simulink model "arq1"  (R2013a)
settings: Solver=ode45  StartTime=0.0  StopTime=Tsim  RelTol=1e-3
values from neighbouring files (symbols this model uses):
  D = 4.1019    [load_variables.m]    (also in matlab.mat; matlab2.mat; matlab_workspace.mat)
  dist = 5    [load_variables.m]    (also in matlab.mat; matlab2.mat; matlab_workspace.mat)
  I = 0.0044    [load_variables.m]    (also in matlab.mat; matlab2.mat; matlab_workspace.mat)
  P = 0.3105    [load_variables.m]    (also in matlab.mat; matlab2.mat; matlab_workspace.mat)
  ref = 10    [load_variables.m]    (also in matlab.mat; matlab2.mat; matlab_workspace.mat)
  Tdist = Tstep    [RenameVar.m]    (also in matlab.mat = 1200; matlab2.mat = 1200; matlab_workspace.mat = 1400)
  Tdistdown = Tstepdown    [RenameVar.m]    (also in matlab.mat = 1800; matlab2.mat = 1800; matlab_workspace.mat = 1800)
  Tref = 800    [load_variables.m]    (also in matlab.mat = 600; matlab2.mat = 600; matlab_workspace.mat = 700)
  Trefdown = Tref+Tstepdown    (= 2420)    [load_variables.m]    (also in matlab.mat = 2400; matlab2.mat = 2400; matlab_workspace.mat = 2500)
  Ts = 5    [load_variables.m]    (also in matlab.mat; matlab2.mat; matlab_workspace.mat)
  Tsim = Tref+Trefdown    (= 3220)    [load_variables.m]    (also in matlab.mat = 800; matlab2.mat = 800; matlab_workspace.mat = 3200)
libraries: opclib x3, simulink x2, commchan3 x1, cstblocks x1
settings Model: Creator=didaticontrol  LastModifiedBy=didaticontrol

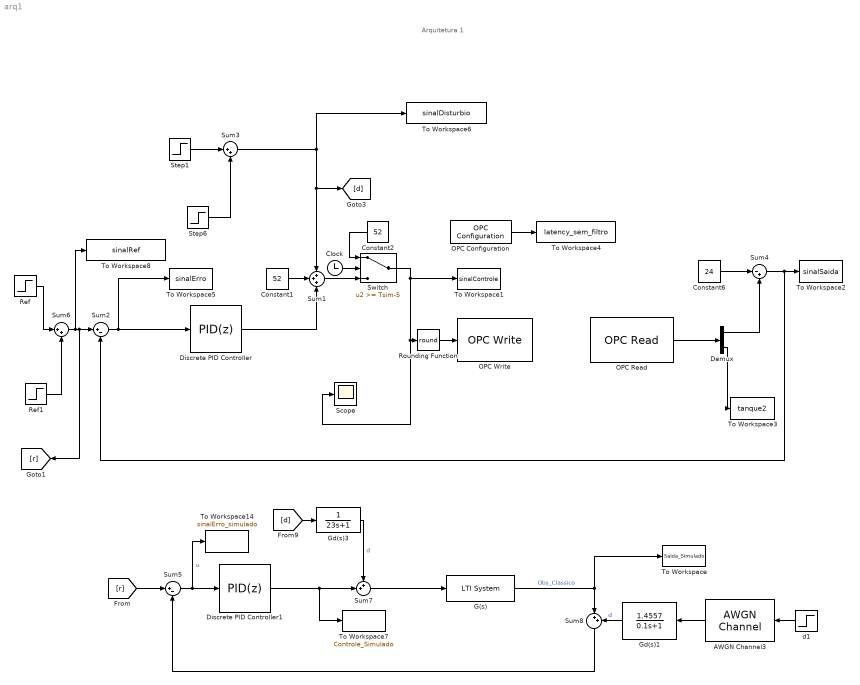
== system arq1 ==
  note: Arquitetura 1
  AWGN Channel3 : commchan3/AWGN Channel  InputProcessing=Columns as channels (frame based)  seed=67  noiseMode=Variance from mask  EbNodB=10  EsNodB=10  SNRdB=10  bitsPerSym=1  Ps=1  Tsym=1  variance=var_ruido
  Clock : Clock
  Constant1 : Constant  Value=52
  Constant2 : Constant  Value=52
  Constant6 : Constant  Value=24
  Demux : Demux  Outputs=2
  Discrete PID Controller : simulink/Continuous/PID Controller  Controller=PID  TimeDomain=Discrete-time  SampleTime=Ts  IntegratorMethod=Forward Euler  FilterMethod=Forward Euler  Form=Parallel  P=P  I=I  D=D  N=0  InitialConditionSource=internal  InitialConditionForIntegrator=0  InitialConditionForFilter=0  ExternalReset=none  LimitOutput=off  UpperSaturationLimit=inf  LowerSaturationLimit=-inf  LinearizeAsGain=off  AntiWindupMode=none  Kb=1  TrackingMode=off  Kt=1  PParamMin=[]  PParamMax=[]  IParamMin=[]  IParamMax=[]  DParamMin=[]  DParamMax=[]  NParamMin=[]  NParamMax=[]  KbParamMin=[]  KbParamMax=[]  KtParamMin=[]  KtParamMax=[]  POutMin=[]  POutMax=[]  IOutMin=[]  IOutMax=[]  DOutMin=[]  DOutMax=[]  NOutMin=[]  NOutMax=[]  KbOutMin=[]  KbOutMax=[]  KtOutMin=[]  KtOutMax=[]  IntegratorOutMin=[]  IntegratorOutMax=[]  FilterOutMin=[]  FilterOutMax=[]  SumOutMin=[]  SumOutMax=[]  SumI1OutMin=[]  SumI1OutMax=[]  SumI2OutMin=[]  SumI2OutMax=[]  SumI3OutMin=[]  SumI3OutMax=[]  SumDOutMin=[]  SumDOutMax=[]  SaturationOutMin=[]  SaturationOutMax=[]  IntegratorContinuousStateAttributes=''  IntegratorStateMustResolveToSignalObject=off  IntegratorRTWStateStorageClass=Auto  FilterContinuousStateAttributes=''  FilterStateMustResolveToSignalObject=off  FilterRTWStateStorageClass=Auto
  Discrete PID Controller1 : simulink/Continuous/PID Controller  Controller=PID  TimeDomain=Discrete-time  SampleTime=Ts  IntegratorMethod=Forward Euler  FilterMethod=Forward Euler  Form=Parallel  P=P  I=I  D=D  N=0  InitialConditionSource=internal  InitialConditionForIntegrator=0  InitialConditionForFilter=0  ExternalReset=none  LimitOutput=off  UpperSaturationLimit=inf  LowerSaturationLimit=-inf  LinearizeAsGain=off  AntiWindupMode=none  Kb=1  TrackingMode=off  Kt=1  PParamMin=[]  PParamMax=[]  IParamMin=[]  IParamMax=[]  DParamMin=[]  DParamMax=[]  NParamMin=[]  NParamMax=[]  KbParamMin=[]  KbParamMax=[]  KtParamMin=[]  KtParamMax=[]  POutMin=[]  POutMax=[]  IOutMin=[]  IOutMax=[]  DOutMin=[]  DOutMax=[]  NOutMin=[]  NOutMax=[]  KbOutMin=[]  KbOutMax=[]  KtOutMin=[]  KtOutMax=[]  IntegratorOutMin=[]  IntegratorOutMax=[]  FilterOutMin=[]  FilterOutMax=[]  SumOutMin=[]  SumOutMax=[]  SumI1OutMin=[]  SumI1OutMax=[]  SumI2OutMin=[]  SumI2OutMax=[]  SumI3OutMin=[]  SumI3OutMax=[]  SumDOutMin=[]  SumDOutMax=[]  SaturationOutMin=[]  SaturationOutMax=[]  IntegratorContinuousStateAttributes=''  IntegratorStateMustResolveToSignalObject=off  IntegratorRTWStateStorageClass=Auto  FilterContinuousStateAttributes=''  FilterStateMustResolveToSignalObject=off  FilterRTWStateStorageClass=Auto
  G(s) : cstblocks/LTI System  sys=Gs  IC=[]
  Gd(s)1 : TransferFcn  Numerator=1.4557  Denominator=[0.1 1]
  Gd(s)3 : TransferFcn  Numerator=1  Denominator=[23 1]
  OPC Configuration : opclib/OPC Configuration  opcServers=143.106.123.105/BR.OPC.Server_AR/10  errMissingItems=Error  errReadWrite=Warn  errShutdown=Error  errRTViolation=Warn  rtEnable=on  speedup=1  showLatency=on  beingUsed=on
  OPC Read : opclib/OPC Read  serverHost=143.106.123.105  serverID=BR.OPC.Server_AR  itemIDs=PTQ4_corrigido, PTQ2_corrigido  readMode=Synchronous (cache)  dataType=double  updateRate=5  showQual=off  showTS=off  tsMode=Seconds since start
  OPC Write : opclib/OPC Write  serverHost=143.106.123.105  serverID=BR.OPC.Server_AR  itemIDs=Bomba2  writeMode=Synchronous  updateRate=-1
  Ref : Step  Time=Tref  After=ref  SampleTime=0
  Ref1 : Step  Time=Trefdown  After=-ref  SampleTime=0
  Rounding Function : Rounding  Operator=round
  Scope : Scope
      settings: YMin=59.0892  YMax=59.0892
  Step1 : Step  Time=Tdist  After=dist  SampleTime=0
  Step6 : Step  Time=Tdistdown  After=-dist  SampleTime=0
  Sum1 : Sum  Inputs=+++
  Sum2 : Sum  Inputs=|+-
  Sum3 : Sum  Inputs=|++
  Sum4 : Sum  Inputs=|-+
  Sum5 : Sum  Inputs=|+-
  Sum6 : Sum  Inputs=|++
  Sum7 : Sum  Inputs=++|
  Sum8 : Sum  Inputs=|++
  Switch : Switch  Threshold=Tsim-5
  To Workspace : ToWorkspace  VariableName=Saida_Simulado  SampleTime=-1  SaveFormat=Timeseries
  To Workspace1 : ToWorkspace  VariableName=sinalControle  SampleTime=Ts  SaveFormat=Timeseries
  To Workspace14 : ToWorkspace  VariableName=sinalErro_simulado  SampleTime=Ts  SaveFormat=Timeseries
  To Workspace2 : ToWorkspace  VariableName=sinalSaida  SampleTime=Ts  SaveFormat=Timeseries
  To Workspace3 : ToWorkspace  VariableName=tanque2  SampleTime=Ts  SaveFormat=Timeseries
  To Workspace4 : ToWorkspace  VariableName=latency_sem_filtro  SampleTime=Ts  SaveFormat=Timeseries
  To Workspace5 : ToWorkspace  VariableName=sinalErro  SampleTime=Ts  SaveFormat=Timeseries
  To Workspace6 : ToWorkspace  VariableName=sinalDisturbio  SampleTime=Ts  SaveFormat=Timeseries
  To Workspace7 : ToWorkspace  VariableName=Controle_Simulado  SampleTime=-1  SaveFormat=Timeseries
  To Workspace8 : ToWorkspace  VariableName=sinalRef  SampleTime=Ts  SaveFormat=Timeseries
  d1 : Step  Time=0  After=0  SampleTime=Ts
  wires:
  Sum2/1 -> To Workspace5/1, Discrete PID Controller/1
  Constant6/1 -> Sum4/1
  Sum4/1 -> Sum2/2, To Workspace2/1
  OPC Read/1 -> Demux/1
  Demux/1 -> Sum4/2
  Demux/2 -> To Workspace3/1
  OPC Configuration/1 -> To Workspace4/1
  Sum3/1 -> [d], Sum1/1, To Workspace6/1
  Step6/1 -> Sum3/2
  Step1/1 -> Sum3/1
  Discrete PID Controller/1 -> Sum1/3
  Constant1/1 -> Sum1/2
  Rounding Function/1 -> OPC Write/1
  [r] -> Sum5/1
  Sum7/1 -> G(s)/1
  G(s)/1 -> To Workspace/1, Sum8/1  "Obs_Classico"
  [d] -> Gd(s)3/1
  Gd(s)3/1 -> Sum7/1  "d"
  Sum8/1 -> Sum5/2
  Sum5/1 -> To Workspace14/1, Discrete PID Controller1/1  "u"
  Discrete PID Controller1/1 -> Sum7/2, To Workspace7/1
  Ref/1 -> Sum6/1
  Ref1/1 -> Sum6/2
  Sum6/1 -> To Workspace8/1, [r], Sum2/1
  Switch/1 -> Scope/1, Rounding Function/1, To Workspace1/1
  Sum1/1 -> Switch/3
  Clock/1 -> Switch/2
  Constant2/1 -> Switch/1
  d1/1 -> AWGN Channel3/1
  AWGN Channel3/1 -> Gd(s)1/1
  Gd(s)1/1 -> Sum8/2  "d"
